simulink model "BMD_2_backup"  (R2025b)
settings: Solver=FixedStepAuto  StartTime=0.0  StopTime=15  FixedStep=0.005  RelTol=1e-3
values from neighbouring files (symbols this model uses):
  FPV_mass = 0.8    [Soft.m]
  g = 9.81    [Soft.m]
  ks = 0    [Soft.m]
  p_0 = 1013.25    [Soft.m]
  Q2Ts = forcetomotors()    [Soft.m]    (also in forcetomotors.m = inv(Ts2Q))
  takeOffDuration = 2    [Soft.m]
  Ts = 0.005    [Soft.m]
undefined symbols (not defined in the file or in its folder): CdA, DiscIntNeverNeededParam, Dw, kd_dz, kd_pos_dx, kd_pos_dy, kd_pq, kd_pr, kd_y, kd_z, ki_dz, ki_pos_dx, ki_pos_dy, ki_pq, ki_pr, ki_y, ki_z, kp_dz, kp_pos_dx, kp_pos_dy, kp_pos_x, kp_pos_y, kp_pq, kp_pr, kp_y, kp_z, pInitialization, rho
libraries: simulink x43, discretizing x18, slpidlib x3, SignalEditorBlockLib x2, shared6dof x1, dynamicsLibrary x1, aerolibasang x1, aerolibnav x1
(part 1 of 22)
settings Model: TunableVars=kd_pq,kd_pr,kd_t,kd_y,ki_pq,ki_pr,ki_t,ki_y,kp_pr,kp_pq,kp_y,kp_t  TunableVarsStorageClass=Auto,Auto,Auto,Auto,Auto,Auto,Auto,Auto,Auto,Auto,Auto,Auto  TunableVarsTypeQualifier=,,,,,,,,,,,  Creator=rafal  LastModifiedBy=rafal
settings OptimizationCC: EnhancedBackFolding=on  PassReuseOutputArgsAs=Individual arguments  ZeroExternalMemoryAtStartup=off  ZeroInternalMemoryAtStartup=off  OptimizeBlockOrder=speed  DifferentSizesBufferReuse=on  OptimizationCustomize=off  EfficientTunableParamExpr=on
settings DebuggingCC: ParameterTunabilityLossMsg=error  BusObjectLabelMismatch=error
settings HardwareCC: ProdBitPerPointer=32.0  ProdBitPerSizeT=32.0  ProdBitPerPtrDiffT=32.0  ProdLargestAtomicInteger=Long  ProdLargestAtomicFloat=Double  ProdWordSize=32.0  ProdHWDeviceType=ARM Compatible->ARM Cortex-M
settings SFSimCC: MATLABDynamicMemAlloc=off
settings RTWCC: SystemTargetFile=ert.tlc  GenCodeOnly=on  TemplateMakefile=ert_default_tmf  Description=Embedded Coder
settings CodeAppCC: ForceParamTrailComments=on  IgnoreCustomStorageClasses=off  OperatorAnnotations=on  SimulinkDataObjDesc=on  SFDataObjDesc=on  InsertBlockDesc=on
settings ERTTargetCC: InlinedParameterPlacement=Hierarchical  ERTCustomFileTemplate=example_file_process.tlc  TargetLangStandard=C99 (ISO)

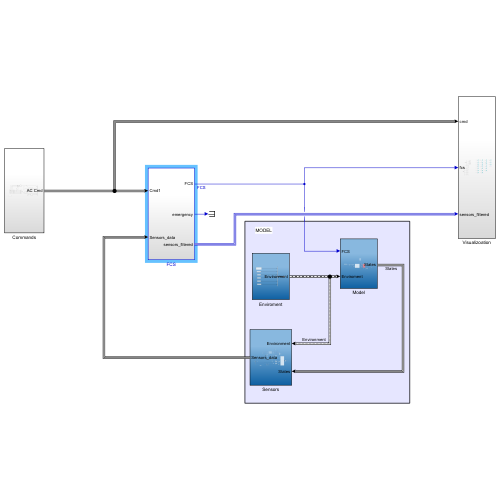
[thumbnail: Simulink's stored preview of the top-level diagram]
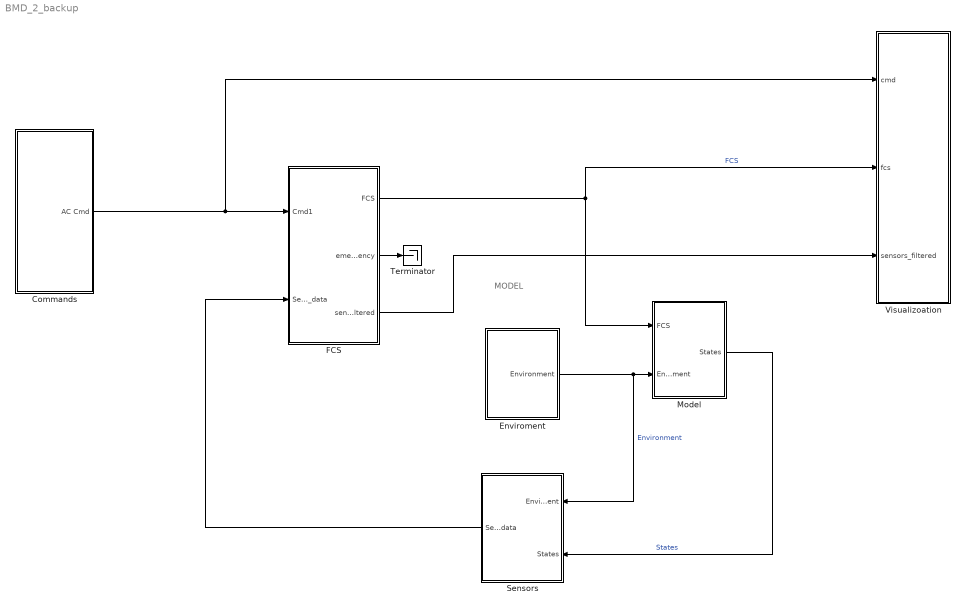
== system BMD_2_backup ==
  note: MODEL
  Commands : Subsystem
  Enviroment : Subsystem
  FCS : Subsystem
  Model : Subsystem
  Sensors : Subsystem
  Terminator : Terminator
  Visualizoation : Subsystem
  wires:
  Enviroment/1(Environment) -> Sensors/1(Environment), Model/2(Enviroment)  "Environment"
  FCS/3(sensors_filtered) -> Visualizoation/3(sensors_filtered)
  FCS/2(emergency) -> Terminator/1
  Model/1(States) -> Sensors/2(States)  "States"
  FCS/1(FCS) -> Model/1(FCS), Visualizoation/2(fcs)  "FCS"
  Sensors/1(Sensors_data) -> FCS/2(Sensors_data)
  Commands/1(AC Cmd) -> FCS/1(Cmd1), Visualizoation/1(cmd)

== system BMD_2_backup/Commands ==
  Bus Creator : BusCreator  Inputs=6  OutDataTypeStr=Bus: CommandBus
  Clock : DigitalClock  SampleTime=0.005
  Clock1 : DigitalClock  SampleTime=0.005
  Compare To Constant : simulink/Logic and Bit Operations/Compare To Constant  relop=<  const=takeOffDuration  OutDataTypeStr=boolean
  Compare To Zero : simulink/Logic and Bit Operations/Compare To Zero  relop===  OutDataTypeStr=uint8
  Compare To Zero1 : simulink/Logic and Bit Operations/Compare To Zero  relop===  OutDataTypeStr=uint8
  Compare To Zero2 : simulink/Logic and Bit Operations/Compare To Zero  relop===  OutDataTypeStr=boolean
  Data Type Conversion1 : DataTypeConversion  OutDataTypeStr=single  SaturateOnIntegerOverflow=off  RndMeth=Floor
  Data Type Conversion2 : DataTypeConversion  OutDataTypeStr=single  SaturateOnIntegerOverflow=off  RndMeth=Floor
  Data Type Conversion3 : DataTypeConversion  OutDataTypeStr=single  SaturateOnIntegerOverflow=off  RndMeth=Floor
  GPS : Subsystem
  Gain : Gain  Gain=1/Ts  OutDataTypeStr=single
  Logical Operator : Logic  Inputs=3  AllPortsSameDT=off  OutDataTypeStr=boolean
  Mux1 : Mux
  Rate Transition{1..4} (4 alike) : RateTransition  OutPortSampleTime=Ts
  Scope : Scope
      settings: ActiveDisplayYMinimum=-1  ActiveDisplayYMaximum=1  DataLoggingVariableName=ScopeData51
  Signal Editor1 : SignalEditorBlockLib/Signal Editor  Commented=on  FileName=signal-test.mat  ActiveScenario=Scenario  ActiveSignal=Signal 1  IsBus=off  OutputBusObjectStr=Bus: BusObject  SampleTime=0  ZeroCross=off  OutputAfterFinalValue=Setting to zero  Unit=inherit  PreserveSignalName=on  ApplySigPropsToAllScenarios=on  ApplySigPropsToAllSignals=off  SignalPropertySource=Dialog parameters
  Step3 : Step  Time=2  Before=1  After=0  SampleTime=0.005  mask(DiscretizedSource){}
      mask init:
      | %zoh
  Step4 : Step  Time=2  After=0  SampleTime=0.005  mask(DiscretizedSource){}
      mask init:
      | %zoh
  Step5 : Step  After=0  SampleTime=0.005  mask(DiscretizedSource){}
      mask init:
      | %zoh
  Step6 : Step  Time=4  Before=1  After=0  SampleTime=0.005  mask(DiscretizedSource){}
      mask init:
      | %zoh
  Transfer Fcn{1..4} (4 alike) : discretizing/Discretized Transfer Fcn  Numerator=[1]  Denominator=[0.08 1]  AbsTol=auto  SampleTime=0.005  method=zoh  Wc=0
  kill_switch : Constant  Value=ks
  AC Cmd : Outport  OutDataTypeStr=Bus: CommandBus  VectorParamsAs1DForOutWhenUnconnected=off
  wires:
  Rate Transition4/1 -> Bus Creator/1  "controlModePosVSOrient"
  Gain/1 -> Bus Creator/5  "live_time_ticks"
  Clock/1 -> Compare To Constant/1
  Rate Transition2/1 -> Bus Creator/2  "pos_ref"
  Mux1/1 -> Data Type Conversion3/1
  Bus Creator/1 -> AC Cmd/1
  Compare To Constant/1 -> Rate Transition3/1
  Step4/1 -> Transfer Fcn2/1, Compare To Zero1/1  "Pitch"
  Data Type Conversion1/1 -> Rate Transition2/1
  Data Type Conversion3/1 -> Rate Transition1/1
  Rate Transition1/1 -> Bus Creator/4  "orient_ref"
  Step5/1 -> Transfer Fcn3/1, Compare To Zero2/1  "Yaw"
  Rate Transition3/1 -> Bus Creator/3  "takeoff_flag"
  Compare To Zero/1 -> Logical Operator/1
  Compare To Zero1/1 -> Logical Operator/2
  Compare To Zero2/1 -> Logical Operator/3
  kill_switch/1 -> Data Type Conversion2/1
  Data Type Conversion2/1 -> Bus Creator/6  "kill_switch"
  Clock1/1 -> Gain/1
  Step3/1 -> Transfer Fcn1/1, Compare To Zero/1  "roll_cmd"
  Transfer Fcn1/1 -> Mux1/1
  Transfer Fcn3/1 -> Mux1/3
  Transfer Fcn4/1 -> Mux1/4
  Transfer Fcn2/1 -> Scope/1, Mux1/2
  Logical Operator/1 -> Rate Transition4/1
  Step6/1 -> Transfer Fcn4/1
  GPS/1(Out1) -> Data Type Conversion1/1

== system BMD_2_backup/Enviroment ==
  Air Density : Constant  Value=1.225  OutDataTypeStr=single
  Air Temp : Constant  Value=288  OutDataTypeStr=single
  Bus Creator : BusCreator  Inputs=6  OutDataTypeStr=Bus: AtmosphereBus  NonVirtualBus=on
  Gravity : Constant  Value=[0 0 9.81]  OutDataTypeStr=single
  Magnetic Field : Constant  Value=[0 0 0]  OutDataTypeStr=single
  Pressure : Constant  Value=1013.25  OutDataTypeStr=single
  Speed of Sound : Constant  Value=340  OutDataTypeStr=single
  Environment : Outport  VectorParamsAs1DForOutWhenUnconnected=off
  wires:
  Magnetic Field/1 -> Bus Creator/6  "MagneticField_ned"
  Air Density/1 -> Bus Creator/5  "air_density"
  Air Temp/1 -> Bus Creator/2  "air_temp"
  Gravity/1 -> Bus Creator/1  "Gravity_ned"
  Speed of Sound/1 -> Bus Creator/3  "speed_sound"
  Bus Creator/1 -> Environment/1
  Pressure/1 -> Bus Creator/4  "pressure"

== system BMD_2_backup/FCS ==
  Cmd1 : Inport  LockScale=on
  Sensors_data : Inport  Port=2
  Bus Selector : BusSelector  OutputSignals=controlModePosVSOrient,orient_ref,takeoff_flag,pos_ref,kill_switch
  Controller : Subsystem
  filters : Subsystem
  value scaling : Subsystem
  FCS : Outport
  emergency : Outport  Port=2
  sensors_filtered : Outport  Port=3
  wires:
  Cmd1/1 -> Bus Selector/1
  Controller/1(FCS) -> FCS/1
  Bus Selector/1 -> Controller/1(In1)  "<controlModePosVSOrient>"
  Bus Selector/3 -> Controller/3(In3)  "<takeoff_flag>"
  Bus Selector/4 -> Controller/4(In4)  "<pos_ref>"
  Sensors_data/1 -> filters/1(Sensors_data)
  filters/1(Sensors_filtered) -> Controller/5(Sensors_filtered), sensors_filtered/1  "sensors_filtered"
  Bus Selector/5 -> emergency/1  "<kill_switch>"
  Bus Selector/2 -> value scaling/1(<orient_ref>)  "<orient_ref>"
  value scaling/1(Out1) -> Controller/2(In2)

== system BMD_2_backup/Model ==
  FCS : Inport
  Enviroment : Inport  Port=2
  6DOF (Quaternion)1 : shared6dof/6DOF (Euler Angles)  units=Metric (MKS)  mtype=Fixed  rep=Euler Angles  xme_0=[0 0 0]  Vm_0=[0 0 0]  eul_0=[0 0 0]  pm_0=[0 0 0]  mass_0=FPV_mass  mass_e=0.5  mass_f=2.0  inertia=diag([0.0016, 0.0022, 0.0035])  inertia_e=eye(3)  inertia_f=2*eye(3)  k_quat=Vehicle.SixDOF.quatGain  vre_flag=on  abi_flag=on  aMode=aMode  xme_statename=''  Vm_statename=''  eul_statename=''  quat_statename=''  pm_statename=''  mass_statename=''
  Abs : Abs  SaturateOnIntegerOverflow=off
  Abs1 : Abs  SaturateOnIntegerOverflow=off
  Add : Sum  Inputs=+++
  Add1 : Sum  Inputs=+++
  Bias1 : Bias  Bias=200  SaturateOnIntegerOverflow=off
  Bus Creator : BusCreator  Inputs=8
  Bus Selector : BusSelector  OutputSignals=air_density
  Constant : Constant  Value=400*[1 1 1 1]
  Data Type Conversion2 : DataTypeConversion  OutDataTypeStr=double  SaturateOnIntegerOverflow=off  RndMeth=Floor
  Data Type Conversion3 : DataTypeConversion  OutDataTypeStr=double  SaturateOnIntegerOverflow=off  RndMeth=Floor
  Gain : Gain  Commented=on  Gain=[1; 1; -1]
  Gain1 : Gain  Gain=(6667 - 200) / 1999
  Gain2 : Gain  Gain=[-1; 1; -1; 1]
  Gain3 : Gain  Gain=-1/2*rho*CdA
  Gain4 : Gain  Gain=-Dw
  Gain5 : Gain  Gain=-[8.0e-3; 8.0e-3; 1.5e-2]
  Gain6 : Gain  Gain=[0; 0; FPV_mass*g]  Multiplication=Matrix(u*K)
  Gain7 : Gain  Gain=g*[0; 0; 1]  Multiplication=Matrix(u*K)
  Gain8 : Gain  Gain=[1 1 -1]
  Gain9 : Gain  Gain=[1 1 -1]
  Minus : Sum  Inputs=+-
  Multirotor : Multirotor  armLength=0.11  CT=0.0168  CQ=1.235e-3  radius=0.0635
  Product1 : Product
  Product2 : Product
  Saturation : Saturate  UpperLimit=4184  LowerLimit=200
  Scope : Scope  NumInputPorts=3
      settings: ActiveDisplayYMinimum=-16.321394872097624  ActiveDisplayYMaximum=12.713488319121959  DataLoggingVariableName=ScopeData11
  Scope1 : Scope
      settings: ActiveDisplayYMinimum=-2.5927814937525517  ActiveDisplayYMaximum=5.2955006788946353  DataLoggingVariableName=ScopeData54
  Scope2 : Scope  NumInputPorts=2
      settings: ActiveDisplayYMinimum=-35.568161441639184  ActiveDisplayYMaximum=36.090415790264551  DataLoggingVariableName=ScopeData31
  Scope3 : Scope  NumInputPorts=2
      settings: ActiveDisplayYMinimum=-3.9266964792505714  ActiveDisplayYMaximum=3.9267975978870897  DataLoggingVariableName=ScopeData64
  Scope4 : Scope
      settings: ActiveDisplayYMinimum=-1  ActiveDisplayYMaximum=1  DataLoggingVariableName=ScopeData56
  Scope8 : Scope
      settings: ActiveDisplayYMinimum=-1  ActiveDisplayYMaximum=1  DataLoggingVariableName=ScopeData41
  Subsystem : Subsystem  Commented=on
  Terminator1 : Terminator
  States : Outport
  wires:
  6DOF (Quaternion)1/1 -> Gain8/1, Bus Creator/1  "V_e"
  6DOF (Quaternion)1/2 -> Bus Creator/2, Gain9/1  "x_e"
  6DOF (Quaternion)1/3 -> Scope3/1, Bus Creator/3  "Euler"
  Bus Creator/1 -> States/1
  6DOF (Quaternion)1/4 -> Gain6/1, Gain7/1, Bus Creator/4  "DCM_be"
  6DOF (Quaternion)1/5 -> Bus Creator/5, Abs/1, Gain3/1  "V_b"
  6DOF (Quaternion)1/6 -> Gain5/1, Gain4/1, Abs1/1, Scope3/2, Bus Creator/6  "omega_b"
  6DOF (Quaternion)1/7 -> Bus Creator/7  "Domega_b"
  6DOF (Quaternion)1/8 -> Scope/2, Minus/1  "Accel_b"
  Subsystem/1(F_xyz) -> Gain/1
  Data Type Conversion3/1 -> Gain1/1
  Enviroment/1 -> Bus Selector/1
  Data Type Conversion2/1 -> Multirotor/2
  Multirotor/1 -> Add/3
  Bias1/1 -> Saturation/1
  Add1/1 -> Scope4/1, 6DOF (Quaternion)1/2
  Bus Selector/1 -> Scope8/1, Data Type Conversion2/1  "<air_density>"
  Gain1/1 -> Bias1/1
  Add/1 -> 6DOF (Quaternion)1/1, Scope1/1
  6DOF (Quaternion)1/9 -> Terminator1/1  "Accel_b"
  Saturation/1 -> Gain2/1
  Gain3/1 -> Product1/2
  Abs/1 -> Product1/1
  Product1/1 -> Add/2
  Multirotor/2 -> Add1/1
  Product2/1 -> Add1/2
  Gain4/1 -> Product2/1
  Abs1/1 -> Product2/2
  Gain5/1 -> Add1/3
  Gain6/1 -> Add/1
  Gain7/1 -> Scope/3, Minus/2
  Minus/1 -> Scope/1, Bus Creator/8  "Accel_b"
  Gain2/1 -> Multirotor/1
  FCS/1 -> Data Type Conversion3/1
  Gain8/1 -> Scope2/2
  Gain9/1 -> Scope2/1

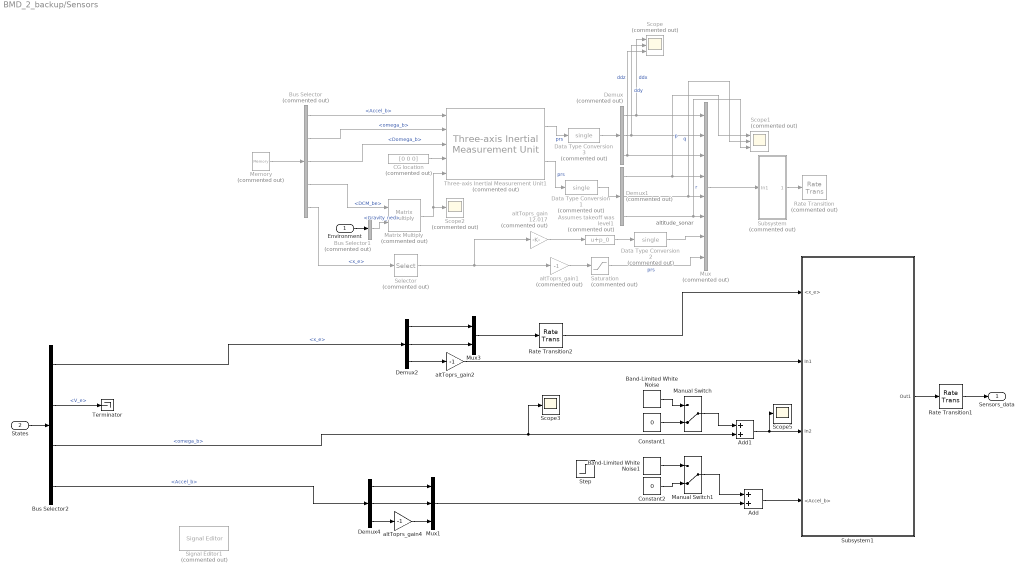
== system BMD_2_backup/Sensors ==
  note: altitude_sonar
  Environment : Inport
  States : Inport  Port=2
  Add : Sum
  Add1 : Sum
  Assumes takeoff was level1 : Bias  Commented=on  Bias=p_0  SaturateOnIntegerOverflow=off
  Band-Limited White Noise : simulink/Sources/Band-Limited White Noise  Cov=[0.000000222]  Ts=0.005  seed=[23341]
  Band-Limited White Noise1 : simulink/Sources/Band-Limited White Noise  Cov=[0.000000222]  Ts=0.005  seed=[23341]
  Bus Selector : BusSelector  Commented=on  OutputSignals=Accel_b,omega_b,Domega_b,DCM_be,x_e
  Bus Selector1 : BusSelector  Commented=on  OutputSignals=Gravity_ned
  Bus Selector2 : BusSelector  OutputSignals=x_e,V_e,omega_b,Accel_b
  CG location : Constant  Commented=on  Value=[0 0 0]
  Constant1 : Constant  Value=0
  Constant2 : Constant  Value=0
  Data Type Conversion1 : DataTypeConversion  Commented=on  OutDataTypeStr=single  SaturateOnIntegerOverflow=off  RndMeth=Floor
  Data Type Conversion2 : DataTypeConversion  Commented=on  OutDataTypeStr=single  SaturateOnIntegerOverflow=off  RndMeth=Floor
  Data Type Conversion3 : DataTypeConversion  Commented=on  OutDataTypeStr=single  SaturateOnIntegerOverflow=off  RndMeth=Floor
  Demux : Demux  Commented=on  Outputs=3
  Demux1 : Demux  Commented=on  Outputs=3
  Demux2 : Demux  Outputs=3
  Demux4 : Demux  Outputs=3
  Manual Switch : ManualSwitch  CurrentSetting=0
  Manual Switch1 : ManualSwitch  CurrentSetting=0
  Matrix Multiply : Product  Commented=on  Multiplication=Matrix(*)
  Memory : Memory  Commented=on
  Mux : Mux  Commented=on  Inputs=8
  Mux1 : Mux  Inputs=3
  Mux3 : Mux  Inputs=2
  Rate Transition : RateTransition  Commented=on
  Rate Transition1 : RateTransition
  Rate Transition2 : RateTransition  OutPortSampleTime=Ts*20
  Saturation : Saturate  Commented=on  UpperLimit=inf  LowerLimit=0  OutDataTypeStr=single
  Scope : Scope  Commented=on  NumInputPorts=3
      settings: ActiveDisplayYMinimum=-74.251567840576172  ActiveDisplayYMaximum=64.477069854736328  DataLoggingVariableName=ScopeData44
  Scope1 : Scope  Commented=on  NumInputPorts=3
      settings: ActiveDisplayYMinimum=-0.22507907450199127  ActiveDisplayYMaximum=0.16993089020252228  DataLoggingVariableName=ScopeData48
  Scope2 : Scope  Commented=on
      settings: ActiveDisplayYMinimum=-1  ActiveDisplayYMaximum=1  DataLoggingVariableName=ScopeData65
  Scope3 : Scope
      settings: ActiveDisplayYMinimum=-1.2738582207061309  ActiveDisplayYMaximum=1.2628218640231634  DataLoggingVariableName=ScopeData5
  Scope5 : Scope
      settings: ActiveDisplayYMinimum=-1.251632855858746  ActiveDisplayYMaximum=1.2544007840477067  DataLoggingVariableName=ScopeData34
  Selector : Selector  Commented=on  InputPortWidth=3  IndexOptions=Index vector (dialog)  Indices=[3]  OutputSizes=1
  Signal Editor1 : SignalEditorBlockLib/Signal Editor  Commented=on  FileName=signal-test.mat  ActiveScenario=Scenario  ActiveSignal=Signal 1  IsBus=off  OutputBusObjectStr=Bus: BusObject  SampleTime=0  ZeroCross=off  OutputAfterFinalValue=Setting to zero  Unit=inherit  PreserveSignalName=on  ApplySigPropsToAllScenarios=on  ApplySigPropsToAllSignals=off  SignalPropertySource=Dialog parameters
  Step : Step  Time=0.1  Before=0.5  SampleTime=0.005  mask(DiscretizedSource){}
      mask init:
      | %zoh
  Subsystem : Subsystem  Commented=on
  Subsystem1 : Subsystem
  Terminator : Terminator
  Three-axis Inertial Measurement Unit1 : aerolibnav/Three-axis Inertial Measurement Unit  Commented=on  units=Metric (MKS)  imu=[0 0 0]  i_Ts=0  dtype_a=on  w_a=190  z_a=0.707  a_sf_cc=[1 0 0; 0 1 0; 0 0 1]  a_bias=[0 0 0]  a_sat="[-inf  -inf  -inf  inf inf inf]"  dtype_g=on  w_g=190  z_g=0.707  g_sf_cc=[1 0 0; 0 1 0; 0 0 1]  g_bias=[0 0 0]  g_sens=[0 0 0]  g_sat="[-inf  -inf  -inf  inf inf inf]"  i_rand=on  i_seeds=[23093 23094 23095 23096 23097 23098]  i_pow=[0.001 0.001 0.001 0.0001 0.0001 0.0001]
  altToprs_gain : Gain  Commented=on  Gain=12.017  ParamDataTypeStr=single  OutDataTypeStr=single
  altToprs_gain1 : Gain  Commented=on  Gain=-1  ParamDataTypeStr=single  OutDataTypeStr=double
  altToprs_gain2 : Gain  Gain=-1  ParamDataTypeStr=single  OutDataTypeStr=double
  altToprs_gain4 : Gain  Gain=-1  ParamDataTypeStr=single  OutDataTypeStr=double
  Sensors_data : Outport
  wires:
  Memory/1 -> Bus Selector/1
  Environment/1 -> Bus Selector1/1
  Bus Selector1/1 -> Matrix Multiply/2  "<Gravity_ned>"
  Bus Selector/4 -> Matrix Multiply/1  "<DCM_be>"
  CG location/1 -> Three-axis Inertial Measurement Unit1/4
  Matrix Multiply/1 -> Scope2/1, Three-axis Inertial Measurement Unit1/5
  Bus Selector/5 -> Selector/1  "<x_e>"
  Bus Selector/3 -> Three-axis Inertial Measurement Unit1/3  "<Domega_b>"
  Bus Selector/2 -> Three-axis Inertial Measurement Unit1/2  "<omega_b>"
  Bus Selector/1 -> Three-axis Inertial Measurement Unit1/1  "<Accel_b>"
  Selector/1 -> altToprs_gain/1, altToprs_gain1/1
  Saturation/1 -> Mux/8  "prs"
  Demux/1 -> Mux/1, Scope/1  "ddx"
  Demux/2 -> Mux/2, Scope/2  "ddy"
  Demux/3 -> Mux/3, Scope/3  "ddz"
  Demux1/1 -> Scope1/1, Mux/4  "p"
  Demux1/2 -> Scope1/2, Mux/5  "q"
  Demux1/3 -> Scope1/3, Mux/6  "r"
  Subsystem/1(Out1) -> Rate Transition/1
  altToprs_gain1/1 -> Saturation/1
  altToprs_gain/1 -> Assumes takeoff was level1/1
  Assumes takeoff was level1/1 -> Data Type Conversion2/1
  Three-axis Inertial Measurement Unit1/1 -> Data Type Conversion3/1  "prs"
  Data Type Conversion3/1 -> Demux/1
  Three-axis Inertial Measurement Unit1/2 -> Data Type Conversion1/1  "prs"
  Data Type Conversion1/1 -> Demux1/1
  Data Type Conversion2/1 -> Mux/7
  Demux2/3 -> altToprs_gain2/1
  Rate Transition1/1 -> Sensors_data/1
  Demux2/2 -> Mux3/2
  Bus Selector2/1 -> Demux2/1  "<x_e>"
  altToprs_gain2/1 -> Subsystem1/2(In1)
  States/1 -> Bus Selector2/1
  Subsystem1/1(Out1) -> Rate Transition1/1
  Demux2/1 -> Mux3/1
  Mux1/1 -> Add/2
  Mux/1 -> Subsystem/1(In1)
  Demux4/1 -> Mux1/1
  Demux4/2 -> Mux1/2
  Demux4/3 -> altToprs_gain4/1
  Bus Selector2/4 -> Demux4/1  "<Accel_b>"
  Add/1 -> Subsystem1/4(<Accel_b>)
  Band-Limited White Noise/1 -> Manual Switch/1
  Add1/1 -> Scope5/1, Subsystem1/3(In2)
  Bus Selector2/2 -> Terminator/1  "<V_e>"
  Manual Switch/1 -> Add1/1
  Band-Limited White Noise1/1 -> Manual Switch1/1
  Manual Switch1/1 -> Add/1
  Constant1/1 -> Manual Switch/2
  altToprs_gain4/1 -> Mux1/3
  Bus Selector2/3 -> Scope3/1, Add1/2  "<omega_b>"
  Constant2/1 -> Manual Switch1/2
  Mux3/1 -> Rate Transition2/1
  Rate Transition2/1 -> Subsystem1/1(<x_e>)

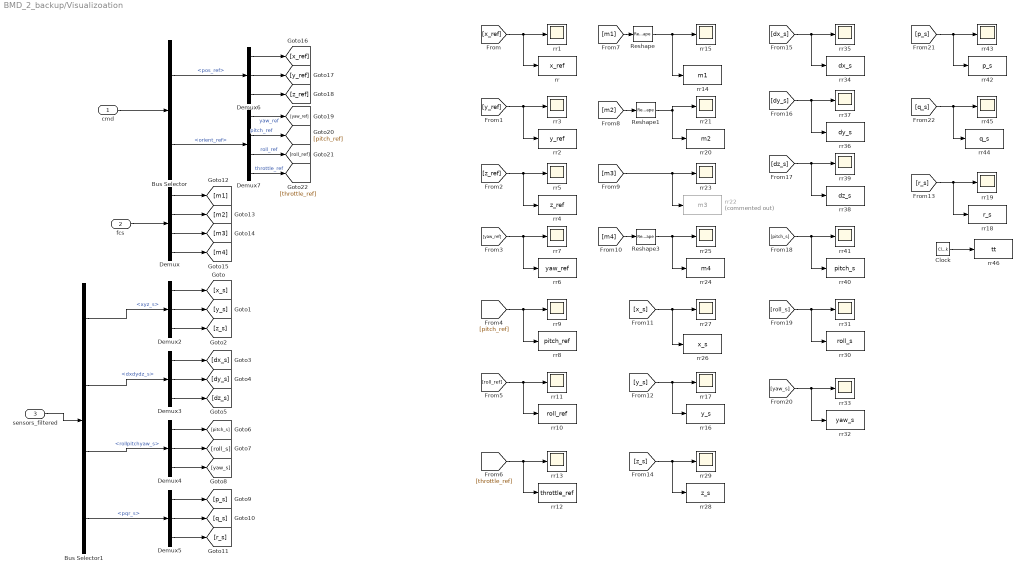
== system BMD_2_backup/Visualizoation ==
  cmd : Inport
  fcs : Inport  Port=2
  sensors_filtered : Inport  Port=3
  Bus Selector : BusSelector  OutputSignals=pos_ref,orient_ref
  Bus Selector1 : BusSelector  OutputSignals=xyz_s,dxdydz_s,rollpitchyaw_s,pqr_s
  Clock : DigitalClock  SampleTime=0.005
  Demux : Demux
  Demux{2..6} (5 alike) : Demux  Outputs=3
  Demux7 : Demux
  Reshape : Reshape
  Reshape1 : Reshape
  Reshape3 : Reshape
  rr : ToWorkspace  VariableName=x_ref  SampleTime=Ts
  rr{1,3,5,7,9,11,13,15,17,19,21,23,25,27,29,31,33,35,37,39,41,43,45} (23 alike) : Scope
      rr1 settings: ActiveDisplayYMinimum=-1  ActiveDisplayYMaximum=1  DataLoggingVariableName=ScopeData10
      rr11 settings: ActiveDisplayYMinimum=-1  ActiveDisplayYMaximum=1  DataLoggingVariableName=ScopeData6
      rr13 settings: ActiveDisplayYMinimum=-1  ActiveDisplayYMaximum=1  DataLoggingVariableName=ScopeData7
      rr15 settings: ActiveDisplayYMinimum=-73.950467746195855  ActiveDisplayYMaximum=1145.5542097157629  DataLoggingVariableName=ScopeData8
      rr17 settings: ActiveDisplayYMinimum=-1  ActiveDisplayYMaximum=1  DataLoggingVariableName=ScopeData9
      rr19 settings: ActiveDisplayYMinimum=-1  ActiveDisplayYMaximum=1  DataLoggingVariableName=ScopeData11
      rr21 settings: ActiveDisplayYMinimum=38  ActiveDisplayYMaximum=58  DataLoggingVariableName=ScopeData12
      rr23 settings: ActiveDisplayYMinimum=-70.597177763307627  ActiveDisplayYMaximum=1115.3745998697689  DataLoggingVariableName=ScopeData13
      rr25 settings: ActiveDisplayYMinimum=46.949385488802776  ActiveDisplayYMaximum=57.45553060077502  DataLoggingVariableName=ScopeData14
      rr27 settings: ActiveDisplayYMinimum=-1  ActiveDisplayYMaximum=1  DataLoggingVariableName=ScopeData15
      rr29 settings: ActiveDisplayYMinimum=-248.57406984307249  ActiveDisplayYMaximum=124.72069577188705  DataLoggingVariableName=ScopeData16
      rr3 settings: ActiveDisplayYMinimum=-5  ActiveDisplayYMaximum=5  DataLoggingVariableName=ScopeData2
      rr31 settings: ActiveDisplayYMinimum=-1  ActiveDisplayYMaximum=1  DataLoggingVariableName=ScopeData17
      rr33 settings: ActiveDisplayYMinimum=-1  ActiveDisplayYMaximum=1  DataLoggingVariableName=ScopeData18
      rr35 settings: ActiveDisplayYMinimum=-1  ActiveDisplayYMaximum=1  DataLoggingVariableName=ScopeData19
      rr37 settings: ActiveDisplayYMinimum=-1  ActiveDisplayYMaximum=1  DataLoggingVariableName=ScopeData20
      rr39 settings: ActiveDisplayYMinimum=-1  ActiveDisplayYMaximum=1  DataLoggingVariableName=ScopeData21
      rr41 settings: ActiveDisplayYMinimum=-1  ActiveDisplayYMaximum=1  DataLoggingVariableName=ScopeData22
      rr43 settings: ActiveDisplayYMinimum=-1  ActiveDisplayYMaximum=1  DataLoggingVariableName=ScopeData23
      rr45 settings: ActiveDisplayYMinimum=-1  ActiveDisplayYMaximum=1  DataLoggingVariableName=ScopeData24
      rr5 settings: ActiveDisplayYMinimum=-1  ActiveDisplayYMaximum=1  DataLoggingVariableName=ScopeData3
      rr7 settings: ActiveDisplayYMinimum=-5  ActiveDisplayYMaximum=5  DataLoggingVariableName=ScopeData4
      rr9 settings: ActiveDisplayYMinimum=-5  ActiveDisplayYMaximum=5  DataLoggingVariableName=ScopeData5
  rr10 : ToWorkspace  VariableName=roll_ref  SampleTime=Ts
  rr12 : ToWorkspace  VariableName=throttle_ref  SampleTime=Ts
  rr14 : ToWorkspace  VariableName=m1  SampleTime=Ts
  rr16 : ToWorkspace  VariableName=y_s  SampleTime=Ts
  rr18 : ToWorkspace  VariableName=r_s  SampleTime=Ts
  rr2 : ToWorkspace  VariableName=y_ref  SampleTime=Ts
  rr20 : ToWorkspace  VariableName=m2  SampleTime=Ts
  rr22 : ToWorkspace  Commented=on  VariableName=m3  SampleTime=Ts
  rr24 : ToWorkspace  VariableName=m4  SampleTime=Ts
  rr26 : ToWorkspace  VariableName=x_s  SampleTime=Ts
  rr28 : ToWorkspace  VariableName=z_s  SampleTime=Ts
  rr30 : ToWorkspace  VariableName=roll_s  SampleTime=Ts
  rr32 : ToWorkspace  VariableName=yaw_s  SampleTime=Ts
  rr34 : ToWorkspace  VariableName=dx_s  SampleTime=Ts
  rr36 : ToWorkspace  VariableName=dy_s  SampleTime=Ts
  rr38 : ToWorkspace  VariableName=dz_s  SampleTime=Ts
  rr4 : ToWorkspace  VariableName=z_ref  SampleTime=Ts
  rr40 : ToWorkspace  VariableName=pitch_s  SampleTime=Ts
  rr42 : ToWorkspace  VariableName=p_s  SampleTime=Ts
  rr44 : ToWorkspace  VariableName=q_s  SampleTime=Ts
  rr46 : ToWorkspace  VariableName=tt  SampleTime=Ts
  rr6 : ToWorkspace  VariableName=yaw_ref  SampleTime=Ts
  rr8 : ToWorkspace  VariableName=pitch_ref  SampleTime=Ts
  wires:
  cmd/1 -> Bus Selector/1
  sensors_filtered/1 -> Bus Selector1/1
  fcs/1 -> Demux/1
  Demux2/3 -> [z_s]
  Demux2/2 -> [y_s]
  Demux2/1 -> [x_s]
  Demux3/3 -> [dz_s]
  Demux3/2 -> [dy_s]
  Demux3/1 -> [dx_s]
  Demux4/3 -> [yaw_s]
  Demux4/2 -> [roll_s]
  Demux4/1 -> [pitch_s]
  Demux5/3 -> [r_s]
  Demux5/2 -> [q_s]
  Demux5/1 -> [p_s]
  Demux/1 -> [m1]
  Demux/4 -> [m4]
  Demux/3 -> [m3]
  Demux/2 -> [m2]
  Demux6/1 -> [x_ref]
  Bus Selector/2 -> Demux7/1  "<orient_ref>"
  Demux7/1 -> [yaw_ref]  "yaw_ref"
  Demux6/3 -> [z_ref]
  Demux7/2 -> [pitch_ref]  "pitch_ref"
  Demux7/3 -> [roll_ref]  "roll_ref"
  Demux6/2 -> [y_ref]
  Bus Selector/1 -> Demux6/1  "<pos_ref>"
  [x_ref] -> rr/1, rr1/1
  Demux7/4 -> [throttle_ref]  "throttle_ref"
  [y_ref] -> rr2/1, rr3/1
  [z_ref] -> rr4/1, rr5/1
  [yaw_ref] -> rr6/1, rr7/1
  [pitch_ref] -> rr8/1, rr9/1
  [roll_ref] -> rr10/1, rr11/1
  [throttle_ref] -> rr12/1, rr13/1
  [y_s] -> rr16/1, rr17/1
  [x_s] -> rr26/1, rr27/1
  [m1] -> Reshape/1
  [m4] -> Reshape3/1
  [r_s] -> rr18/1, rr19/1
  [roll_s] -> rr30/1, rr31/1
  [dx_s] -> rr34/1, rr35/1
  [dy_s] -> rr36/1, rr37/1
  [pitch_s] -> rr40/1, rr41/1
  [z_s] -> rr28/1, rr29/1
  [dz_s] -> rr38/1, rr39/1
  [yaw_s] -> rr32/1, rr33/1
  [p_s] -> rr42/1, rr43/1
  [q_s] -> rr44/1, rr45/1
  Bus Selector1/1 -> Demux2/1  "<xyz_s>"
  Bus Selector1/2 -> Demux3/1  "<dxdydz_s>"
  Bus Selector1/3 -> Demux4/1  "<rollpitchyaw_s>"
  Bus Selector1/4 -> Demux5/1  "<pqr_s>"
  Clock/1 -> rr46/1
  Reshape/1 -> rr14/1, rr15/1
  [m2] -> Reshape1/1
  [m3] -> rr22/1, rr23/1
  Reshape3/1 -> rr24/1, rr25/1
  Reshape1/1 -> rr21/1, rr20/1

== system BMD_2_backup/Commands/GPS ==
  Mux2 : Mux  Inputs=3
  Step : Step  After=0  SampleTime=0.005  mask(DiscretizedSource){}
      mask init:
      | %zoh
  Step1 : Step  After=0  SampleTime=0.005  mask(DiscretizedSource){}
      mask init:
      | %zoh
  Step2 : Step  After=0  SampleTime=0.005  mask(DiscretizedSource){}
      mask init:
      | %zoh
  Transfer Fcn5 : discretizing/Discretized Transfer Fcn  Numerator=[1]  Denominator=[0.08 1]  AbsTol=auto  SampleTime=0.005  method=zoh  Wc=0
  Transfer Fcn6 : discretizing/Discretized Transfer Fcn  Numerator=[1]  Denominator=[0.08 1]  AbsTol=auto  SampleTime=0.005  method=zoh  Wc=0
  Transfer Fcn7 : discretizing/Discretized Transfer Fcn  Numerator=[1]  Denominator=[0.08 1]  AbsTol=auto  SampleTime=0.005  method=zoh  Wc=0
  Out1 : Outport
  wires:
  Transfer Fcn5/1 -> Mux2/1
  Mux2/1 -> Out1/1
  Step1/1 -> Transfer Fcn6/1
  Step/1 -> Transfer Fcn5/1
  Transfer Fcn6/1 -> Mux2/2
  Transfer Fcn7/1 -> Mux2/3
  Step2/1 -> Transfer Fcn7/1

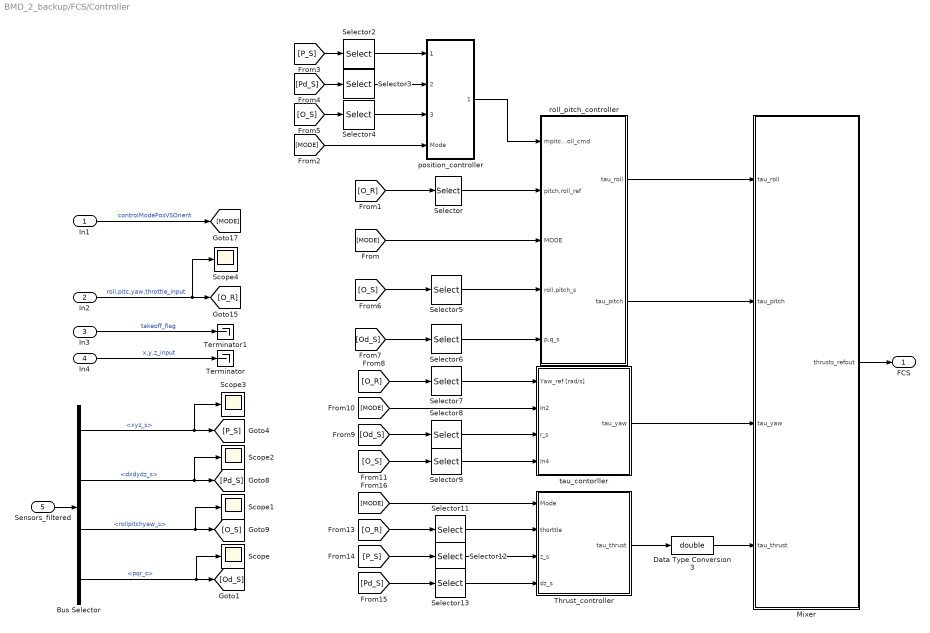
== system BMD_2_backup/FCS/Controller ==
  In1 : Inport
  In2 : Inport  Port=2
  In3 : Inport  Port=3
  In4 : Inport  Port=4
  Sensors_filtered : Inport  Port=5
  Bus Selector : BusSelector  OutputSignals=xyz_s,dxdydz_s,rollpitchyaw_s,pqr_s
  Data Type Conversion3 : DataTypeConversion  OutDataTypeStr=double  SaturateOnIntegerOverflow=off  RndMeth=Floor
  Mixer : Subsystem
  Scope{,1..4} (5 alike) : Scope
      Scope settings: ActiveDisplayYMinimum=-1  ActiveDisplayYMaximum=1  DataLoggingVariableName=ScopeData26
      Scope1 settings: ActiveDisplayYMinimum=-1  ActiveDisplayYMaximum=1  DataLoggingVariableName=ScopeData27
      Scope2 settings: ActiveDisplayYMinimum=-1  ActiveDisplayYMaximum=1  DataLoggingVariableName=ScopeData28
      Scope3 settings: ActiveDisplayYMinimum=-198.01537047970481  ActiveDisplayYMaximum=949.36258849660373  DataLoggingVariableName=ScopeData29
      Scope4 settings: ActiveDisplayYMinimum=-0.61312502622604359  ActiveDisplayYMaximum=5.5181252360343933  DataLoggingVariableName=ScopeData30
  Selector : Selector  InputPortWidth=4  IndexOptions=Index vector (dialog)  Indices=[1 2]  OutputSizes=1
  Selector11 : Selector  InputPortWidth=4  IndexOptions=Index vector (dialog)  Indices=[4]  OutputSizes=1
  Selector{4,8..9,12..13} (5 alike) : Selector  InputPortWidth=3  IndexOptions=Index vector (dialog)  Indices=[3]  OutputSizes=1
  Selector{2..3,5..6} (4 alike) : Selector  InputPortWidth=3  IndexOptions=Index vector (dialog)  Indices=[1 2]  OutputSizes=1
  Selector7 : Selector  InputPortWidth=4  IndexOptions=Index vector (dialog)  Indices=[3]  OutputSizes=1
  Terminator : Terminator
  Terminator1 : Terminator
  Thrust_controller : Subsystem
  position_controller : Subsystem
  roll_pitch_controller : Subsystem
  tau_contorller : Subsystem
  FCS : Outport
  wires:
  Mixer/1(thrusts_refout) -> FCS/1
  In1/1 -> [MODE]  "controlModePosVSOrient"
  In2/1 -> Scope4/1, [O_R]  "roll,pitc,yaw,throttle_input"
  In3/1 -> Terminator1/1  "takeoff_flag"
  In4/1 -> Terminator/1  "x,y,z_input"
  Sensors_filtered/1 -> Bus Selector/1
  Bus Selector/2 -> Scope2/1, [Pd_S]  "<dxdydz_s>"
  Bus Selector/1 -> Scope3/1, [P_S]  "<xyz_s>"
  roll_pitch_controller/1(tau_roll) -> Mixer/1(tau_roll)
  tau_contorller/1(tau_yaw) -> Mixer/3(tau_yaw)
  Bus Selector/4 -> Scope/1, [Od_S]  "<pqr_s>"
  Bus Selector/3 -> Scope1/1, [O_S]  "<rollpitchyaw_s>"
  [P_S] -> Selector2/1
  [Pd_S] -> Selector3/1
  Selector2/1 -> position_controller/1(x,y,_s)
  Selector3/1 -> position_controller/2(dx,dy_s)
  [O_S] -> Selector4/1
  Selector4/1 -> position_controller/3(yaw_s)
  [O_S] -> Selector5/1
  [Od_S] -> Selector6/1
  Selector5/1 -> roll_pitch_controller/4(roll,pitch_s)
  Selector6/1 -> roll_pitch_controller/5(p,q_s)
  Selector8/1 -> tau_contorller/3(r_s)
  [Od_S] -> Selector8/1
  [O_R] -> Selector11/1
  Selector12/1 -> Thrust_controller/3(z_s)
  Selector13/1 -> Thrust_controller/4(dz_s)
  [P_S] -> Selector12/1
  [Pd_S] -> Selector13/1
  [MODE] -> Thrust_controller/1(Mode)
  [O_R] -> Selector7/1
  [MODE] -> tau_contorller/2(In2)
  Selector7/1 -> tau_contorller/1(Yaw_ref [rad/s])
  [O_R] -> Selector/1
  Selector/1 -> roll_pitch_controller/2(pitch,roll_ref)
  [MODE] -> roll_pitch_controller/3(MODE)
  Selector11/1 -> Thrust_controller/2(thorttle)
  roll_pitch_controller/2(tau_pitch) -> Mixer/2(tau_pitch)
  Data Type Conversion3/1 -> Mixer/4(tau_thrust)
  [O_S] -> Selector9/1
  Selector9/1 -> tau_contorller/4(In4)
  Thrust_controller/1(tau_thrust) -> Data Type Conversion3/1
  [MODE] -> position_controller/4(Mode)
  position_controller/1(pitch_roll_cmd) -> roll_pitch_controller/1(mpitch_roll_cmd)

== system BMD_2_backup/FCS/filters ==
  Sensors_data : Inport  OutDataTypeStr=Bus: sensors_mes
  Bus Creator : BusCreator  Inputs=4  OutDataTypeStr=Bus: Sensors_filtered
  Bus Selector : BusSelector  OutputSignals=timestamp_ms,status,GPS_s,axayaz_s,pqr_sf,pressure_s,mxmymz_s,altitude_s,temp_s,vbat_s
  Data Type Conversion1 : DataTypeConversion  OutDataTypeStr=single  SaturateOnIntegerOverflow=off  RndMeth=Floor
  Data Type Conversion3 : DataTypeConversion  OutDataTypeStr=single  SaturateOnIntegerOverflow=off  RndMeth=Floor
  LPF_altitude : discretizing/Discretized Transfer Fcn  Numerator=[1]  Denominator=[1 1]  AbsTol=auto  SampleTime=0.005  method=zoh  Wc=0
  Subsystem : Subsystem
  Subsystem1 : Subsystem
  Terminator{,1..5} (6 alike) : Terminator
  Transfer Fcn : discretizing/Discretized Transfer Fcn  Numerator=[1]  Denominator=[0.1 1]  AbsTol=auto  SampleTime=0.005  method=zoh  Wc=0
  Transfer Fcn2 : discretizing/Discretized Transfer Fcn  Numerator=[1]  Denominator=[0.1 1]  AbsTol=auto  SampleTime=0.005  method=zoh  Wc=0
  pqr_LPF1 : Subsystem
  pqr_LPF2 : Subsystem
  Sensors_filtered : Outport
  wires:
  Bus Selector/1 -> Terminator/1  "<timestamp_ms>"
  Bus Selector/2 -> Terminator1/1  "<status>"
  Bus Selector/10 -> Terminator3/1  "<vbat_s>"
  Bus Selector/7 -> Transfer Fcn2/1  "<mxmymz_s>"
  Bus Selector/8 -> LPF_altitude/1  "<altitude_s>"
  Bus Selector/9 -> Transfer Fcn/1  "<temp_s>"
  LPF_altitude/1 -> [B]  "pressure_f"
  Bus Selector/6 -> Terminator2/1  "<pressure_s>"
  Transfer Fcn/1 -> Terminator4/1  "temp_f"
  Transfer Fcn2/1 -> Terminator5/1  "alt_f"
  [B] -> Subsystem/2(pressure_f)  "pressure_f"
  Subsystem/1(x,y,z) -> Bus Creator/1  "xyz_s"
  Subsystem/2(dx,dy,dz) -> Bus Creator/2  "dxdydz_s"
  Subsystem1/1(orient_earth) -> Subsystem/4(orient_earth), Bus Creator/3  "rollpitchyaw_s"
  Bus Creator/1 -> Sensors_filtered/1
  Sensors_data/1 -> Bus Selector/1
  pqr_LPF1/1(ax,ay,az) -> Data Type Conversion3/1  "ax,ay,ax_f"
  Bus Selector/5 -> pqr_LPF2/1(p,q,r)  "<pqr_sf>"
  Data Type Conversion1/1 -> Bus Creator/4, Subsystem1/2(p,q,r_f)  "pqr_s"
  pqr_LPF2/1(p,q,r_f) -> Data Type Conversion1/1  "pqr_s"
  Bus Selector/4 -> pqr_LPF1/1(1)  "<axayaz_s>"
  Data Type Conversion3/1 -> Subsystem1/1(ax,ay,ax_f), Subsystem/3(ax,ay,ax_f)
  Bus Selector/3 -> Subsystem/1(GPS_s)  "<GPS_s>"

== system BMD_2_backup/FCS/value scaling ==
  <orient_ref> : Inport
  Dead Zone : DeadZone  LowerValue=-0.03  UpperValue=0.03
  Demux : Demux
  Gain : Gain  Gain=0.5236  ParamDataTypeStr=single
  Gain1 : Gain  Gain=0.5236  OutDataTypeStr=single
  Gain2 : Gain  Gain=0.5236  OutDataTypeStr=single
  Gain3 : Gain  Gain=(FPV_mass*g)-0.5  OutDataTypeStr=single
  Mux : Mux
  Saturation{1..4} (4 alike) : Saturate  UpperLimit=1  LowerLimit=-1
  Out1 : Outport
  wires:
  Mux/1 -> Out1/1
  <orient_ref>/1 -> Dead Zone/1
  Demux/2 -> Saturation2/1  "pitch"
  Demux/1 -> Saturation1/1  "roll"
  Demux/3 -> Saturation3/1  "yaw"
  Demux/4 -> Saturation4/1  "throttle"
  Gain/1 -> Mux/1  "<-0.5236;0.5236> [Rad]"
  Gain1/1 -> Mux/2  "<-0.5236;0.5236> [Rad]"
  Dead Zone/1 -> Demux/1
  Saturation1/1 -> Gain/1
  Saturation2/1 -> Gain1/1
  Saturation3/1 -> Gain2/1
  Gain2/1 -> Mux/3  "<-0.5236;0.5236> [Rad/s]"
  Gain3/1 -> Mux/4  "<-4.905;4.905> [N]"
  Saturation4/1 -> Gain3/1

== system BMD_2_backup/Model/Subsystem ==
  FCS : Inport
  Enviroment : Inport  Port=2
  DCM(angeles) : Inport  Port=3
  V_b : Inport  Port=4
  omega_b : Inport  Port=5
  Add : Sum  Inputs=+++
  Add1 : Sum  Inputs=++++
  Bus Selector : BusSelector  OutputSignals=Gravity_ned,air_density
  Constant : Constant  Value=0
  Constant1 : Constant  Value=0
  Data Type Conversion{1..5} (5 alike) : DataTypeConversion  OutDataTypeStr=double  SaturateOnIntegerOverflow=off  RndMeth=Floor
  Demux : Demux
  Gain{,1..3} (4 alike) : Gain  Gain=6.0/1999
  Manual Switch : ManualSwitch  CurrentSetting=0
  Motor Forces and Torques : Subsystem
  Mux : Mux  Inputs=3
  Saturation : Saturate  UpperLimit=25  LowerLimit=-25  OutDataTypeStr=double
  Scope : Scope  NumInputPorts=3
      settings: ActiveDisplayYMinimum=-0.000142277817061181  ActiveDisplayYMaximum=0.00017675284388450334  DataLoggingVariableName=ScopeData69
  Scope1 : Scope
      settings: ActiveDisplayYMinimum=-1  ActiveDisplayYMaximum=1  DataLoggingVariableName=ScopeData71
  Scope2 : Scope
      settings: ActiveDisplayYMinimum=-1.3749999694671553  ActiveDisplayYMaximum=12.3749997252044  DataLoggingVariableName=ScopeData69
  drag forces : Subsystem
  gravity forces : Subsystem
  F_xyz : Outport
  m_xyz : Outport  Port=2
  wires:
  Add/1 -> Saturation/1
  Bus Selector/1 -> Data Type Conversion1/1  "<Gravity_ned>"
  Enviroment/1 -> Bus Selector/1
  DCM(angeles)/1 -> gravity forces/2(DCM(angeles))
  gravity forces/1(Out1) -> Scope/1, Add/1
  drag forces/1(Out1) -> Add/2, Scope/2
  Bus Selector/2 -> Data Type Conversion3/1  "<air_density>"
  V_b/1 -> Scope1/1, Data Type Conversion2/1
  omega_b/1 -> Data Type Conversion4/1
  FCS/1 -> Data Type Conversion5/1
  Motor Forces and Torques/1(Motor Forces) -> Scope/3, Add/3
  Motor Forces and Torques/2(Motor Torques) -> m_xyz/1
  Saturation/1 -> Manual Switch/1
  Data Type Conversion3/1 -> drag forces/1(pressure), Motor Forces and Torques/2(Density)
  Data Type Conversion1/1 -> gravity forces/1(gravity)
  Data Type Conversion2/1 -> Motor Forces and Torques/1(Vb), drag forces/2(V_b)
  Data Type Conversion4/1 -> Motor Forces and Torques/3(pqr)
  Data Type Conversion5/1 -> Demux/1, Motor Forces and Torques/4(Motor Commands)
  Manual Switch/1 -> Scope2/1, F_xyz/1
  Mux/1 -> Manual Switch/2
  Constant/1 -> Mux/1
  Constant1/1 -> Mux/2
  Demux/1 -> Gain/1
  Demux/2 -> Gain1/1
  Demux/4 -> Gain3/1
  Demux/3 -> Gain2/1
  Gain3/1 -> Add1/4
  Gain2/1 -> Add1/3
  Gain1/1 -> Add1/2
  Gain/1 -> Add1/1
  Add1/1 -> Mux/3

== system BMD_2_backup/Sensors/Subsystem ==
  In1 : Inport
  Bus Creator : BusCreator  Inputs=9  OutDataTypeStr=Bus: sensors_mes
  Demux : Demux  Outputs=8
  Mux1 : Mux  Inputs=3
  Mux2 : Mux  Inputs=3
  Subsystem : Subsystem
  Zero{,1..3} (4 alike) : Constant  Value=0  OutDataTypeStr=single
  Out1 : Outport
  wires:
  In1/1 -> Demux/1
  Zero/1 -> Bus Creator/1  "timestamp_ms"
  Zero1/1 -> Bus Creator/2  "status"
  Mux1/1 -> Bus Creator/3  "axayaz_s"
  Mux2/1 -> Bus Creator/4  "pqr_sf"
  Subsystem/1(Out1) -> Bus Creator/5  "mxmymz_s"
  Demux/1 -> Mux1/1
  Demux/2 -> Mux1/2
  Demux/3 -> Mux1/3
  Demux/4 -> Mux2/1
  Demux/5 -> Mux2/2
  Demux/6 -> Mux2/3
  Demux/7 -> Bus Creator/6  "altitude_s"
  Demux/8 -> Bus Creator/7  "pressure_s"
  Zero2/1 -> Bus Creator/8  "temp_s"
  Zero3/1 -> Bus Creator/9  "vbat_s"
  Bus Creator/1 -> Out1/1

== system BMD_2_backup/Sensors/Subsystem1 ==
  <x_e> : Inport
  In1 : Inport  Port=2
  In2 : Inport  Port=3
  <Accel_b> : Inport  Port=4
  Add : Sum
  Band-Limited White Noise1 : simulink/Sources/Band-Limited White Noise  Cov=[0.004]  Ts=0.1  seed=[23341]
  Bus Creator : BusCreator  Inputs=10  OutDataTypeStr=Bus: sensors_mes
  Constant : Constant  Value=0
  Data Type Conversion{1..4} (4 alike) : DataTypeConversion  OutDataTypeStr=single  SaturateOnIntegerOverflow=off  RndMeth=Floor
  Manual Switch1 : ManualSwitch  CurrentSetting=0
  Scope : Scope
      settings: ActiveDisplayYMinimum=-0.62920108548628406  ActiveDisplayYMaximum=0.75699628484534132  DataLoggingVariableName=ScopeData38
  Subsystem : Subsystem
  Zero{,1..4} (5 alike) : Constant  Value=0  OutDataTypeStr=single
  Out1 : Outport
  wires:
  Zero/1 -> Bus Creator/1  "timestamp_ms"
  Zero1/1 -> Bus Creator/2  "status"
  Subsystem/1(Out1) -> Bus Creator/6  "mxmymz_s"
  Zero2/1 -> Bus Creator/9  "temp_s"
  Zero3/1 -> Bus Creator/10  "vbat_s"
  Bus Creator/1 -> Out1/1
  Zero4/1 -> Bus Creator/8  "pressure_s"
  Data Type Conversion3/1 -> Bus Creator/7  "altitude_s"
  Data Type Conversion2/1 -> Bus Creator/4  "axayaz_s"
  Data Type Conversion1/1 -> Bus Creator/5  "pqr_sf"
  In1/1 -> Add/2  "altitude_s"
  In2/1 -> Data Type Conversion1/1  "pqr_sf"
  <Accel_b>/1 -> Data Type Conversion2/1  "axayaz_s"
  Band-Limited White Noise1/1 -> Manual Switch1/1
  Constant/1 -> Manual Switch1/2
  Manual Switch1/1 -> Add/1, Scope/1
  Add/1 -> Data Type Conversion3/1
  <x_e>/1 -> Data Type Conversion4/1
  Data Type Conversion4/1 -> Bus Creator/3  "GPS_s"

== system BMD_2_backup/FCS/Controller/Mixer ==
  tau_roll : Inport
  tau_pitch : Inport  Port=2
  tau_yaw : Inport  Port=3
  tau_thrust : Inport  Port=4
  Matrix Multiply : Product  Commented=on  Multiplication=Matrix(*)
  Multiply : Gain  Gain=Q2Ts  Multiplication=Matrix(K*u)
  Mux : Mux
  Reshape : Reshape  Commented=on  OutputDimensionality=Customize  OutputDimensions=[4,1]
  Reshape1 : Reshape  OutputDimensionality=Customize  OutputDimensions=[4,1]
  Saturation : Saturate  UpperLimit=9.0  LowerLimit=0.15
  Saturation5 : Saturate  UpperLimit=2047  LowerLimit=48
  ThrustToMotorCommand : Gain  Gain=(2047-48)/9.0  OutDataTypeStr=single
  TorqueTotalThrustToThrustPerMotor : Constant  Commented=on  Value=Q2Ts  OutDataTypeStr=single
  Transpose : Math  Commented=on  Operator=transpose
  thrusts_refout : Outport
  wires:
  Mux/1 -> Reshape1/1
  Multiply/1 -> Saturation/1
  Saturation5/1 -> thrusts_refout/1
  ThrustToMotorCommand/1 -> Saturation5/1
  TorqueTotalThrustToThrustPerMotor/1 -> Matrix Multiply/1
  Reshape/1 -> Matrix Multiply/2
  tau_thrust/1 -> Mux/1
  tau_roll/1 -> Mux/2
  tau_pitch/1 -> Mux/3
  tau_yaw/1 -> Mux/4
  Reshape1/1 -> Multiply/1
  Saturation/1 -> ThrustToMotorCommand/1

== system BMD_2_backup/FCS/Controller/Thrust_controller ==
  Mode : Inport
  thorttle : Inport  Port=2
  z_s : Inport  Port=3
  dz_s : Inport  Port=4
  Compare To Constant1 : simulink/Logic and Bit Operations/Compare To Constant  relop===  const=0  OutDataTypeStr=boolean
  Constant : Constant  Value=g*FPV_mass  OutDataTypeStr=single
  Constant2 : Constant  Value=0
  Discrete-Time Integrator : DiscreteIntegrator  gainval=0.6  ExternalReset=level  SampleTime=0.005  LimitOutput=on  UpperSaturationLimit=1.5  LowerSaturationLimit=-1.5  ICPrevOutput=DiscIntNeverNeededParam  ICPrevScaledInput=DiscIntNeverNeededParam
  Gain : Gain  Gain=0.6
  Kd_z : Gain  Gain=kd_z
  PID Controller (2DOF) : slpidlib/PID Controller (2DOF)  Controller=PID  Form=Parallel  TimeDomain=Discrete-time  UseExternalTs=off  SampleTime=0.005  IntegratorMethod=Forward Euler  FilterMethod=Forward Euler  ControllerParametersSource=internal  P=kp_dz  I=ki_dz  UseKiTs=off  D=kd_dz  UseExternalDerivativeSource=off  N=50  UseFilter=on  b=1  c=1  TunerSelectOption=Transfer Function Based (PID Tuner App)  InitialConditionSource=internal  InitialConditionForIntegrator=0  InitialConditionForFilter=0  DifferentiatorICPrevScaledInput=0  ExternalReset=none  TrackingMode=on  Kt=1  LimitOutput=on  SatLimitsSource=internal  UpperSaturationLimit=10.0  LowerSaturationLimit=-4.5  LinearizeAsGain=on  AntiWindupMode=clamping  Kb=1  LimitIntegrator=on  UpperIntegratorSaturationLimit=4.9  LowerIntegratorSaturationLimit=-4.9  RndMeth=Ceiling  PGainOutDataTypeStr=single  PProdOutDataTypeStr=single  POutMin=[]  POutMax=[]  IGainOutDataTypeStr=single  IProdOutDataTypeStr=single  IOutMin=[]  IOutMax=[]  DGainOutDataTypeStr=single  DProdOutDataTypeStr=single  DOutMin=[]  DOutMax=[]  NGainOutDataTypeStr=single  NProdOutDataTypeStr=single  NOutMin=[]  NOutMax=[]  bGainOutDataTypeStr=single  bProdOutDataTypeStr=single  bOutMin=[]  bOutMax=[]  cGainOutDataTypeStr=single  cProdOutDataTypeStr=single  cOutMin=[]  cOutMax=[]  SumOutDataTypeStr=single  SumOutMin=[]  SumOutMax=[]  SaturationOutMin=[]  SaturationOutMax=[]  PParamDataTypeStr=single  PParamMin=[]  PParamMax=[]  IParamDataTypeStr=single  IParamMin=[]  IParamMax=[]  DParamDataTypeStr=single  DParamMin=[]  DParamMax=[]  NParamDataTypeStr=single  NParamMin=[]  NParamMax=[]  bParamDataTypeStr=single  bParamMin=[]  bParamMax=[]  cParamDataTypeStr=single  cParamMin=[]  cParamMax=[]  KbParamMin=[]  KbParamMax=[]  KtParamMin=[]  KtParamMax=[]  KbOutMin=[]  KbOutMax=[]  KtOutMin=[]  KtOutMax=[]  IntegratorOutMin=[]  IntegratorOutMax=[]  FilterOutMin=[]  FilterOutMax=[]  SumI1OutMin=[]  SumI1OutMax=[]  SumI2OutMin=[]  SumI2OutMax=[]  SumI3OutMin=[]  SumI3OutMax=[]  SumI4OutMin=[]  SumI4OutMax=[]  SumDOutDataTypeStr=single  SumDOutMin=[]  SumDOutMax=[]  Sum1OutDataTypeStr=single  Sum1OutMin=[]  Sum1OutMax=[]  Sum2OutDataTypeStr=single  Sum2OutMin=[]  Sum2OutMax=[]  Sum3OutDataTypeStr=single  Sum3OutMin=[]  Sum3OutMax=[]  SumAccumDataTypeStr=single  SumDAccumDataTypeStr=single  Sum1AccumDataTypeStr=single  Sum2AccumDataTypeStr=single  Sum3AccumDataTypeStr=single  DifferentiatorOutMin=[]  DifferentiatorOutMax=[]  FilterDiffOutCoefMin=[]  FilterDiffOutCoefMax=[]  ReciprocalOutMin=[]  ReciprocalOutMax=[]  SumDenOutMin=[]  SumDenOutMax=[]  SumNumOutMin=[]  SumNumOutMax=[]  DivideOutMin=[]  DivideOutMax=[]  UdiffTsProdOutMin=[]  UdiffTsProdOutMax=[]  NTsProdOutMin=[]  NTsProdOutMax=[]  UintegralTsProdOutMin=[]  UintegralTsProdOutMax=[]  UngainTsProdOutMin=[]  UngainTsProdOutMax=[]  ClampingZeroOutDataTypeStr=Inherit: Inherit via back propagation  ClampingZeroOutMin=[]  ClampingZeroOutMax=[]  FilterDenConstantOutDataTypeStr=Inherit: Inherit via back propagation  FilterDenConstantOutMin=[]  FilterDenConstantOutMax=[]  PCopyOutDataTypeStr=Inherit: Inherit via back propagation  PCopyOutMin=[]  PCopyOutMax=[]  NCopyOutDataTypeStr=single  NCopyOutMin=[]  NCopyOutMax=[]  IntegratorContinuousStateAttributes=''  IntegratorStateMustResolveToSignalObject=off  IntegratorRTWStateStorageClass=Auto  FilterContinuousStateAttributes=''  FilterStateMustResolveToSignalObject=off  FilterRTWStateStorageClass=Auto  ParallelPVariant=InternalParameters  IdealPVariant=Disabled  IVariant=InternalParameters  DVariant=InternalParameters  bVariant=InternalParameters  cVariant=InternalParameters  IntegratorVariant=Discrete  SatVariant=Enabled  AWVariant=DiscClampingParallel  PCopyVariant=Disabled  TRVariant=Enabled  FdbkBlocksVariant=Forward  IdealPFdbkVariant=Disabled  SatFdbkVariant=Disabled  DerivativeFilterVariant=ForwardEulerFilter  NVariant=InternalParameters  NCopyVariant=Disabled  FilterICVariant=InternalICsFilter  IntegratorICVariant=InternalICs  ExternalResetVariant=Disabled  TRSumVariant=TrackingMode  SumFdbkVariant=Disabled  SumVariant=Sum_PID  TsampFilterVariant=InternalTs  TsampNgainVariant=Passthrough  TsampIntegralVariant=Disabled_SignalSpec  ExternalSaturationOutDataTypeStr=Inherit: Same as second input  DerivativeSourceVariant=ErrorSignal  PreIntVariant=InternalPreInt
  Power_thrust : Gain  Gain=0.8
  Saturation1 : Saturate  UpperLimit=10.0  LowerLimit=0.2
  Saturation_dz : Saturate  UpperLimit=15.0  LowerLimit=-15.0
  Saturation_z : Saturate  UpperLimit=15.0  LowerLimit=-15.0
  Sum : Sum  Inputs=++|
  Sum1 : Sum  Inputs=++|
  Sum3 : Sum  Inputs=+-|
  Sum4 : Sum  Inputs=+|+|+
  Switch : Switch  Criteria=u2 > Threshold  SaturateOnIntegerOverflow=off  InputSameDT=off
  Switch1 : Switch  Criteria=u2 > Threshold  SaturateOnIntegerOverflow=off  InputSameDT=off
  Switch2 : Switch  Criteria=u2 > Threshold  OutDataTypeStr=single  SaturateOnIntegerOverflow=off  InputSameDT=off
  Switch3 : Switch  Criteria=u2 > Threshold  SaturateOnIntegerOverflow=off  InputSameDT=off
  Terminator1 : Terminator
  Unit Delay : UnitDelay  SampleTime=-1  HasFrameUpgradeWarning=on
  Unit Delay1 : UnitDelay  SampleTime=-1  HasFrameUpgradeWarning=on
  ki_z : Gain  Gain=ki_z  OutDataTypeStr=single
  kp_z : Gain  Gain=kp_z  OutDataTypeStr=single
  tau_thrust : Outport
  wires:
  Switch2/1 -> Sum1/2  "wynik"
  Switch/1 -> Switch2/1
  Sum3/1 -> ki_z/1, kp_z/1
  kp_z/1 -> Sum4/2
  Discrete-Time Integrator/1 -> Sum4/3
  ki_z/1 -> Discrete-Time Integrator/1
  Unit Delay/1 -> Switch3/1
  Sum/1 -> Sum3/1  "wysokosc_ref"
  Sum4/1 -> Saturation_z/1  "pid"
  Constant2/1 -> Switch/3
  Saturation1/1 -> tau_thrust/1
  Constant/1 -> Sum1/1
  z_s/1 -> Sum3/2, Switch3/3  "wysokosc"
  Mode/1 -> Terminator1/1
  Gain/1 -> Sum/1
  Sum1/1 -> Saturation1/1
  Switch1/1 -> Gain/1, Unit Delay1/1
  Compare To Constant1/1 -> Switch3/2, Switch1/2, Discrete-Time Integrator/2, Switch/2, Switch2/2
  Unit Delay1/1 -> Switch1/1
  Switch3/1 -> Unit Delay/1, Sum/2
  PID Controller (2DOF)/1 -> Saturation_dz/1
  Saturation_z/1 -> PID Controller (2DOF)/1
  dz_s/1 -> Switch1/3, Kd_z/1, PID Controller (2DOF)/2
  thorttle/1 -> PID Controller (2DOF)/3, Power_thrust/1, Compare To Constant1/1
  Kd_z/1 -> Sum4/1
  Power_thrust/1 -> Switch2/3
  Saturation_dz/1 -> Switch/1
